simulink model "ddm"  (R2021a)
settings: Solver=ode4  StartTime=0.0  StopTime=2  FixedStep=0.01  RelTol=1e-3
values from neighbouring files (symbols this model uses):
  d = 800 + 400 * rand(nsim,1)    [monte_parsim.m]
  k = 9000    [monte_parsim.m]
  m = 450    [monte_parsim.m]
  s0 = 0    [monte_parsim.m]
  v0 = 0.1    [monte_parsim.m]
settings Model: Creator=ceanb  LastModifiedBy=ceanb

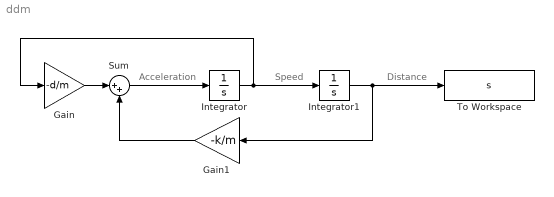
== system ddm ==
  note: Acceleration
  note: Speed
  note: Distance
  Gain : Gain  Gain=-d/m
  Gain1 : Gain  Gain=-k/m
  Integrator : Integrator  InitialCondition=v0
  Integrator1 : Integrator  InitialCondition=s0
  Sum : Sum  Inputs=|++
  To Workspace : ToWorkspace  VariableName=s  SampleTime=-1
      settings: Save2DSignal=2-D array (concatenate along first dimension)
  wires:
  Integrator/1 -> Gain/1, Integrator1/1
  Sum/1 -> Integrator/1
  Gain/1 -> Sum/1
  Integrator1/1 -> To Workspace/1, Gain1/1
  Gain1/1 -> Sum/2
